simulink model "exercise01"  (R2022a)
settings: Solver=VariableStepAuto  StartTime=0.0  StopTime=20  RelTol=1e-3
settings Model: Creator=ac133867  LastModifiedBy=cunis
settings DebuggingCC: UnconnectedInputMsg=warning  UnconnectedOutputMsg=warning  UnconnectedLineMsg=warning
settings RTWCC: DLArmComputeVersion=19.05

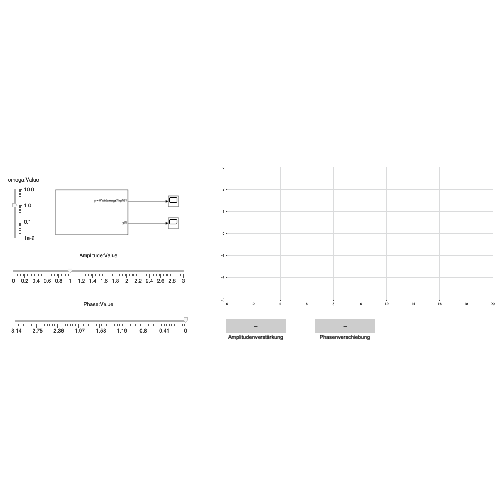
[thumbnail: Simulink's stored preview of the top-level diagram]
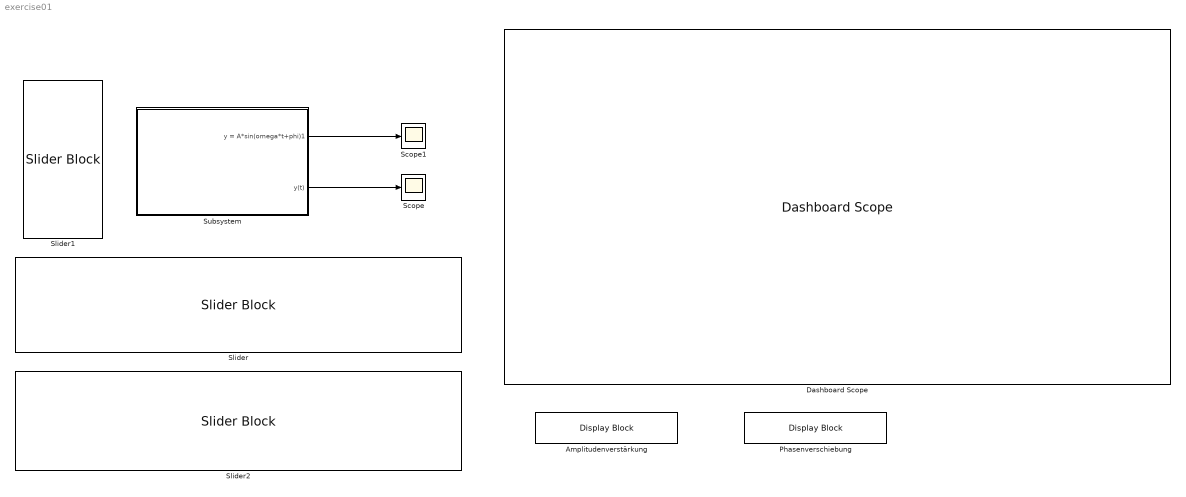
== system exercise01 ==
  Amplitudenverstärkung : DisplayBlock  LabelPosition=Hide  Format=Custom  Transparency=1  FormatString=A = %0.3g
  Dashboard Scope : DashboardScope
  Phasenverschiebung : DisplayBlock  LabelPosition=Hide  Format=Custom  Transparency=1  FormatString=phi = %0.3g
  Scope : Scope
  Scope1 : Scope
  Slider : SliderBlock  ScaleMax=3
  Slider1 : SliderBlock  ScaleMin=0.01  ScaleMax=10  ScaleType=Log
  Slider2 : SliderBlock  ScaleMin=-3.14  ScaleMax=0
  Subsystem : Subsystem
  wires:
  Subsystem/1(y = A*sin(omega*t+phi)1) -> Scope1/1
  Subsystem/2(y(t)) -> Scope/1

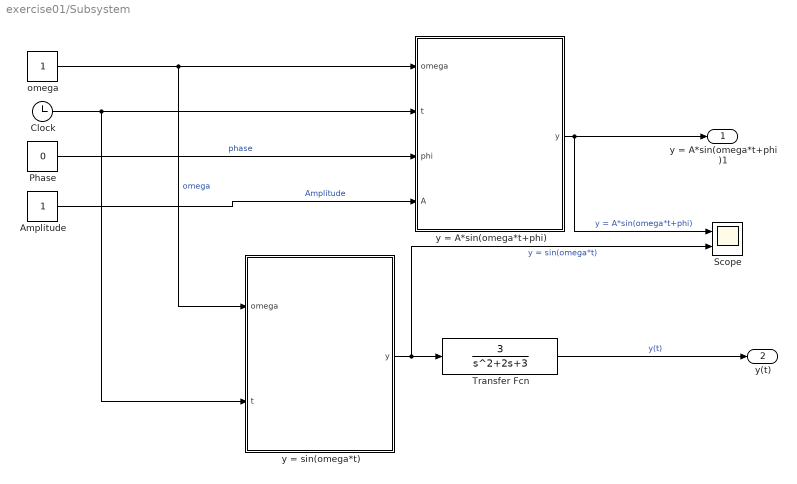
== system exercise01/Subsystem ==
  Amplitude : Constant
  Clock : Clock
  Phase : Constant  Value=0
  Scope : Scope  NumInputPorts=2
  Transfer Fcn : TransferFcn  Numerator=[3]  Denominator=[1 2 3]
  omega : Constant
  y = A*sin(omega*t+phi) : MATLAB Function  TreatAsAtomicUnit=on
  y = sin(omega*t) : MATLAB Function  TreatAsAtomicUnit=on
  y = A*sin(omega*t+phi)1 : Outport
  y(t) : Outport  Port=2
  wires:
  omega/1 -> y = sin(omega*t)/1(omega), y = A*sin(omega*t+phi)/1(omega)  "omega"
  Clock/1 -> y = sin(omega*t)/2(t), y = A*sin(omega*t+phi)/2(t)
  y = A*sin(omega*t+phi)/1(y) -> Scope/1, y = A*sin(omega*t+phi)1/1  "y = A*sin(omega*t+phi)"
  y = sin(omega*t)/1(y) -> Scope/2, Transfer Fcn/1  "y = sin(omega*t)"
  Amplitude/1 -> y = A*sin(omega*t+phi)/4(A)  "Amplitude"
  Transfer Fcn/1 -> y(t)/1  "y(t)"
  Phase/1 -> y = A*sin(omega*t+phi)/3(phi)  "phase"

== matlab function exercise01/Subsystem/y = sin(omega*t) ==
  data: omega input; t input; y output
function y = fcn(omega, t)


y = sin(omega*t);

== matlab function exercise01/Subsystem/y = A*sin(omega*t+phi) ==
  data: omega input; t input; y output; phi input; A input
function y = fcn(omega, t, phi,A)


y = A*sin(omega*t+phi);
